simulink model "trottinette"  (R2020a)
settings: Solver=VariableStepAuto  StartTime=0.0  StopTime=10.0  RelTol=1e-3
libraries: cstblocks x3
settings Model: Creator=siard  LastModifiedBy=siard

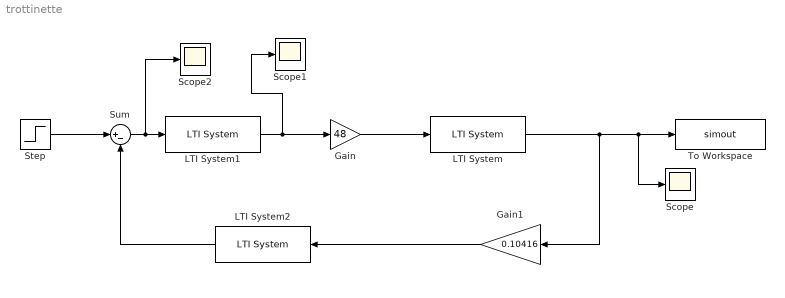
== system trottinette ==
  Gain : Gain  Gain=48
  Gain1 : Gain  Gain=0.10416
  LTI System : cstblocks/LTI System  sys=Gm  IC=[]
  LTI System1 : cstblocks/LTI System  sys=C  IC=[]
  LTI System2 : cstblocks/LTI System  sys=F  IC=[]
  Scope : Scope
  Scope1 : Scope
  Scope2 : Scope
  Step : Step  After=1.65  SampleTime=0
  Sum : Sum  Inputs=|+-
  To Workspace : ToWorkspace  VariableName=simout  SaveFormat=Timeseries  SampleTime=-1
  wires:
  Sum/1 -> Scope2/1, LTI System1/1
  LTI System2/1 -> Sum/2
  LTI System/1 -> Gain1/1, Scope/1, To Workspace/1
  Gain/1 -> LTI System/1
  Gain1/1 -> LTI System2/1
  Step/1 -> Sum/1
  LTI System1/1 -> Scope1/1, Gain/1
